simulink model "matprob3"  (R2020a)
settings: Solver=VariableStepAuto  StartTime=0.0  StopTime=10.0  RelTol=1e-3
libraries: simulink x1
settings Model: Creator=deepa  LastModifiedBy=deepa

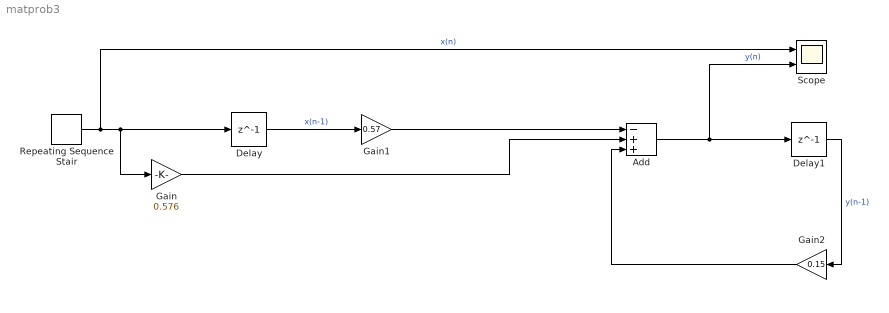
== system matprob3 ==
  Add : Sum  Inputs=-++
  Delay : Delay  DelayLength=1
  Delay1 : Delay  DelayLength=1
  Gain : Gain  Gain=0.576
  Gain1 : Gain  Gain=0.57
  Gain2 : Gain  Gain=0.15
  Repeating Sequence Stair : simulink/Sources/Repeating Sequence Stair  OutValues=[3 1 4 2 1].'  tsamp=-1  OutMin=[]  OutMax=[]  OutDataTypeStr=double  OutputDataTypeScalingMode=double  OutDataType=fixdt(0,8)  ConRadixGroup=Best Precision: Vector-wise  OutScaling=2^-12
  Scope : Scope  NumInputPorts=2
  wires:
  Repeating Sequence Stair/1 -> Scope/1, Gain/1, Delay/1  "x(n)"
  Delay/1 -> Gain1/1  "x(n-1)"
  Gain1/1 -> Add/1
  Gain/1 -> Add/2
  Add/1 -> Scope/2, Delay1/1  "y(n)"
  Delay1/1 -> Gain2/1  "y(n-1)"
  Gain2/1 -> Add/3
